simulink model "LAB3_CrazyFlie_2024_245678987654"  (R2023b)
settings: Solver=ode45  StartTime=0.0  StopTime=inf  MaxStep=0.1  RelTol=1e-3  EnableMultiTasking=on
PreLoadFcn:
  | % load parameters of the default quadrotor
  | disp('Quadrotor parameters loaded by PreLoadFcn')
  | mdl_quadrotor
values from neighbouring files (symbols this model uses):
  x = pos(:, 1)    [lab3_trajectory.m]    (also in plot.m = timeseries(x, time))
  y = pos(:, 2)    [lab3_trajectory.m]    (also in plot.m = timeseries(y, time))
  yaw = atan2(-y, -x)    [lab3_trajectory.m]    (also in plot.m = timeseries(yaw, time))
  z = pos(:, 3)    [lab3_trajectory.m]    (also in plot.m = timeseries(z, time))
undefined symbols (not defined in the file or in its folder): angdiff, Angular, Linear, rot2
libraries: robotlib x3, simulink x1
settings Model: Creator=corkep  LastModifiedBy=hampu
settings SolverCC: AlgebraicLoopSolver=TrustRegion
settings DataIOCC: LimitDataPoints=on  ReturnWorkspaceOutputs=off
settings OptimizationCC: ReuseModelBlockBuffer=off  ExpressionDepthLimit=2147483647  LifeSpan=inf
settings DebuggingCC: UnderspecifiedInitializationDetection=Classic  MergeDetectMultiDrivingBlocksExec=none  SolverPrmCheckMsg=warning  UnconnectedInputMsg=warning  UnconnectedOutputMsg=warning  UnconnectedLineMsg=warning  AllowSymbolicDim=off  StateNameClashWarn=warning  SFUnexpectedBacktrackingDiag=warning  SFNoUnconditionalDefaultTransitionDiag=warning  SFExecutionAtInitializationDiag=none  ArithmeticOperatorsInVariantConditions=warning
settings HardwareCC: ProdBitPerPointer=32  ProdBitPerSizeT=32  ProdBitPerPtrDiffT=32  ProdLargestAtomicFloat=None  ProdIntDivRoundTo=Undefined  ProdEndianess=Unspecified  ProdWordSize=32  ProdHWDeviceType=32-bit Generic
settings ModelReferenceCC: EnableRefExpFcnMdlSchedulingChecks=on  PropagateSignalLabelsOutOfModel=off
settings SFSimCC: SimUseLocalCustomCode=off  CustomCodeUndefinedFunction=UseInterfaceOnly
settings RTWCC: RTWUseLocalCustomCode=off  DLArmComputeVersion=19.05
settings CodeAppCC: StateflowObjectComments=on
settings GRTTargetCC: TargetLangStandard=C89/C90 (ANSI)  CombineOutputUpdateFcns=off  GRTInterface=on
settings ConfigComp: CovMetricSettings=dw  CovSaveCumulativeToWorkspaceVar=on  CovSaveSingleToWorkspaceVar=on  CovExternalEMLEnable=off  CovSFcnEnable=off

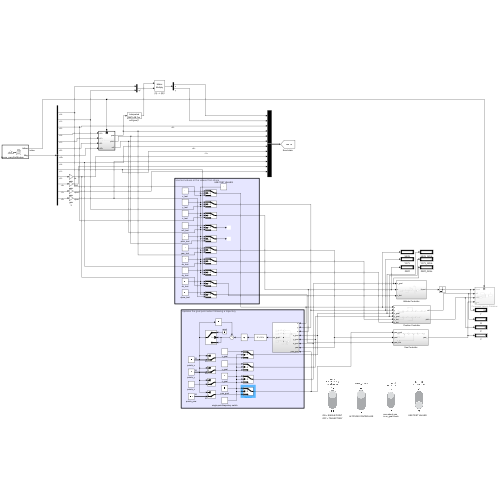
[thumbnail: Simulink's stored preview of the top-level diagram]
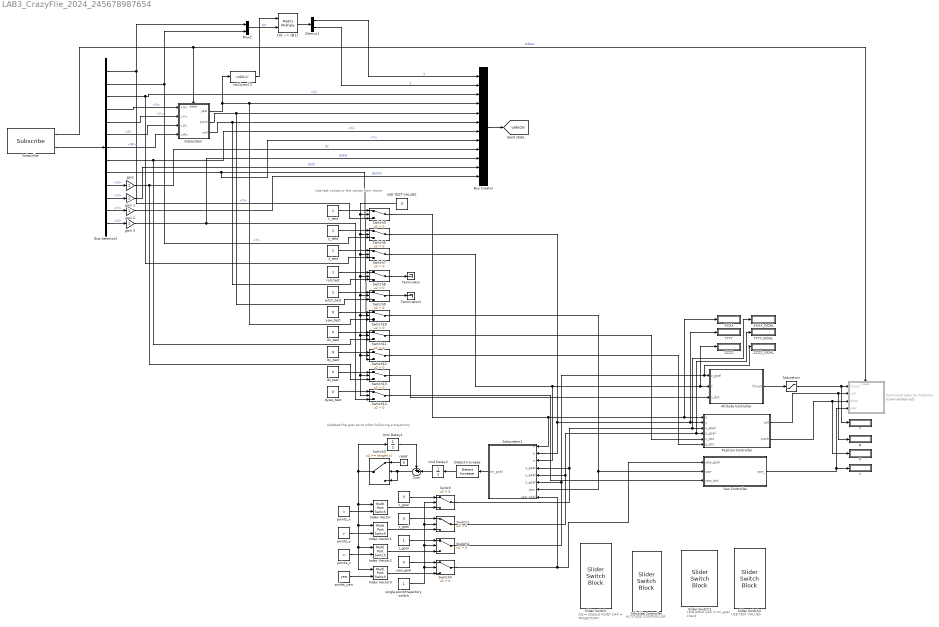
== system LAB3_CrazyFlie_2024_245678987654 ==
  note: Use test values or the values from drone
  note: USE TEST VALUES
  note: care about yaw
      | in on_goal check
  note: ON = SINGLE POINT
      | OFF = TRAJECTORY
  note: Updates the goal point when following a trajectory
  note: ALTITUDE CONTROLLER
  Altitude Controller : Subsystem
  Altiutide Controller : SliderSwitchBlock
      settings: Values={{'Off', 'On'}, [0 1]}
  Bus Creator : BusCreator  Inputs=12
  Bus Selector3 : BusSelector  OutputSignals=Pose.Pose.Position.X,Pose.Pose.Position.Y,Pose.Pose.Position.Z,Pose.Pose.Orientation.X,Pose.Pose.Orientation.Y,Pose.Pose.Orientation.Z,Pose.Pose.Orientation.W,Twist.Twist.Linear.X,Twist.Twist.Linear.Y,Twist.Twist.Linear.Z,Twist.Twist.Angular.X,Twist.Twist.Angular.Y,Twist.Twist.Angular.Z
  Command Velocity Publisher : Subsystem  Commented=on
  Demux1 : Demux  Outputs=2
  Detect Increase : simulink/Logic and Bit Operations/Detect Increase  vinit=0.0  OutDataTypeStr=boolean
  Index Vector{,1..3} (4 alike) : MultiPortSwitch  DataPortOrder=Zero-based contiguous  Inputs=1  zeroidx=on  SaturateOnIntegerOverflow=off  InputSameDT=off
  Mux2 : Mux  Inputs=2
  P : Display
  Position Controller : Subsystem
  R : Display
  Saturation : Saturate  UpperLimit=1  LowerLimit=0
  Slider Switch : SliderSwitchBlock
      settings: Values={{'Off', 'On'}, [0 1]}
  Slider Switch1 : SliderSwitchBlock
      settings: Values={{'Off', 'On'}, [0 1]}
  Slider Switch2 : SliderSwitchBlock
      settings: Values={{'Off', 'On'}, [0 1]}
  Subscribe : robotlib/Subscribe  topicSource=Select from ROS network  topic=/pixy/vicon/demo_crazyflie28/demo_crazyflie28/odom  messageType=nav_msgs/Odometry  SampleTime=-1  legacyBusStruct=off  messageQueueLength=51
  Subsystem : Subsystem
  Subsystem1 : Subsystem
  Sum : Sum  Inputs=++|
  Switch{,1..2,4..14} (14 alike) : Switch  Criteria=u2 > Threshold  SaturateOnIntegerOverflow=off  InputSameDT=off
  Switch3 : Switch  Threshold=length(x)  SaturateOnIntegerOverflow=off  InputSameDT=off
  T : Display
  Terminator : Terminator
  Terminator1 : Terminator
  USE TEST VALUES : Constant  Value=0
  Unit Delay2 : UnitDelay  SampleTime=-1  HasFrameUpgradeWarning=on
  Unit Delay4 : UnitDelay  SampleTime=-1  HasFrameUpgradeWarning=on
  XXXX : Display
  XXXX_GOAL : Display
  Y : Display
  YYYY : Display
  YYYY_GOAL : Display
  Yaw Controller : Subsystem
  ZZZZ : Display
  ZZZZ_GOAL : Display
  dx_test : Constant  Value=0
  dy_test : Constant  Value=0
  dyaw_test : Constant  Value=0
  dz_test : Constant  Value=0
  gain {,1..3} (4 alike) : Gain
  pitch_test : Constant
  points_x : Constant  Value=x
  points_y : Constant  Value=y
  points_yaw : Constant  Value=yaw
  points_z : Constant  Value=z
  reset : Constant  Value=0  VectorParams1D=off
  roll_test : Constant
  rot2(yaw)'1 : MATLABFcn  MATLABFcn=rot2(u)'  OutputDimensions=[2 2]  Output1D=off
  single point/trajectory switch : Constant
  x_goal : Constant  Value=3
  x_test : Constant
  y_goal : Constant  Value=3
  y_test : Constant
  yaw_goal : Constant  Value=0
  yaw_test : Constant  Value=0
  z_goal : Constant
  z_test : Constant
  "{0} --> {B}1" : Product  Multiplication=Matrix(*)  RndMeth=Zero
  tag scope: vehicle=global
  wires:
  Bus Selector3/11 -> gain 1/1  "<X>"
  Bus Selector3/13 -> gain 3/1  "<Z>"
  Bus Selector3/10 -> "gain "/1  "<Z>"
  Bus Selector3/9 -> Switch12/3, Bus Creator/8  "<Y>"
  Bus Selector3/8 -> Switch11/3, Bus Creator/7  "<X>"
  Bus Selector3/3 -> Switch7/3, Bus Creator/3  "<Z>"
  Bus Creator/1 -> [vehicle]
  Bus Selector3/12 -> gain 2/1  "<Y>"
  Subscribe/2 -> Bus Selector3/1
  Subscribe/1 -> Subsystem/Enable, Command Velocity Publisher/Enable  "IsNew"
  Mux2/1 -> "{0} --> {B}1"/2  "xy*"
  "{0} --> {B}1"/1 -> Demux1/1
  Demux1/1 -> Bus Creator/1  "x"
  Demux1/2 -> Bus Creator/2  "y"
  Bus Selector3/1 -> Mux2/1, Switch5/3  "<X>"
  Bus Selector3/2 -> Switch6/3, Mux2/2  "<Y>"
  rot2(yaw)'1/1 -> "{0} --> {B}1"/1
  "gain "/1 -> Switch13/3, Bus Creator/9  "dz"
  gain 1/1 -> Bus Creator/11  "droll"
  gain 2/1 -> Bus Creator/12  "dpitch"
  gain 3/1 -> Switch14/3, Bus Creator/10  "dyaw"
  Subsystem/1(yaw) -> rot2(yaw)'1/1, Switch10/3, Bus Creator/4
  Bus Selector3/4 -> Subsystem/1(<X>)  "<X>"
  Bus Selector3/5 -> Subsystem/2(<Y>)  "<Y>"
  Bus Selector3/6 -> Subsystem/3(<Z>)  "<Z>"
  Bus Selector3/7 -> Subsystem/4(<W>)  "<W>"
  Subsystem/2(pitch) -> Switch9/3, Bus Creator/5
  Subsystem/3(roll) -> Switch8/3, Bus Creator/6
  Altitude Controller/1(thrust) -> Saturation/1
  Saturation/1 -> T/1, Command Velocity Publisher/1(thrust)
  x_goal/1 -> Switch/1
  Position Controller/2(pitch) -> P/1, Command Velocity Publisher/3(pitch)
  Position Controller/1(roll) -> R/1, Command Velocity Publisher/2(roll)
  Yaw Controller/1(yaw_) -> Command Velocity Publisher/4(yaw), Y/1
  Unit Delay4/1 -> Sum/1
  Sum/1 -> Switch3/3, Switch3/2
  Unit Delay2/1 -> Sum/2
  Switch3/1 -> Index Vector3/1, Index Vector2/1, Index Vector1/1, Index Vector/1, Unit Delay4/1
  reset/1 -> Switch3/1
  Detect Increase/1 -> Unit Delay2/1
  Subsystem1/1(on_goal) -> Detect Increase/1
  points_x/1 -> Index Vector/2
  points_y/1 -> Index Vector1/2
  points_z/1 -> Index Vector2/2
  points_yaw/1 -> Index Vector3/2
  Switch/1 -> XXXX_GOAL/1, Position Controller/3(x_goal), Subsystem1/4(x_goal)
  Index Vector/1 -> Switch/3
  Index Vector1/1 -> Switch1/3
  Index Vector2/1 -> Switch2/3
  Index Vector3/1 -> Switch4/3
  y_goal/1 -> Switch1/1
  z_goal/1 -> Switch2/1
  yaw_goal/1 -> Switch4/1
  single point/trajectory switch/1 -> Switch/2, Switch1/2, Switch2/2, Switch4/2
  Switch4/1 -> Subsystem1/8(yaw_goal), Yaw Controller/1(yaw_goal)
  Switch2/1 -> ZZZZ_GOAL/1, Altitude Controller/1(z_goal), Subsystem1/6(z_goal)
  Switch1/1 -> YYYY_GOAL/1, Position Controller/4(y_goal), Subsystem1/5(y_goal)
  x_test/1 -> Switch5/1
  y_test/1 -> Switch6/1
  z_test/1 -> Switch7/1
  USE TEST VALUES/1 -> Switch14/2, Switch13/2, Switch12/2, Switch11/2, Switch10/2, Switch9/2, Switch8/2, Switch7/2, Switch6/2, Switch5/2
  roll_test/1 -> Switch8/1
  pitch_test/1 -> Switch9/1
  yaw_test/1 -> Switch10/1
  dx_test/1 -> Switch11/1
  dy_test/1 -> Switch12/1
  dz_test/1 -> Switch13/1
  dyaw_test/1 -> Switch14/1
  Switch7/1 -> Subsystem1/3(z), ZZZZ/1, Altitude Controller/2(z)
  Switch5/1 -> XXXX/1, Position Controller/1(x), Subsystem1/1(x)
  Switch6/1 -> YYYY/1, Position Controller/2(y), Subsystem1/2(y)
  Switch8/1 -> Terminator/1
  Switch10/1 -> Subsystem1/7(yaw), Yaw Controller/2(yaw)
  Switch11/1 -> Position Controller/5(x_dot)
  Switch12/1 -> Position Controller/6(y_dot)
  Switch13/1 -> Altitude Controller/3(z_dot)
  Switch14/1 -> Yaw Controller/3(yaw_dot)
  Switch9/1 -> Terminator1/1

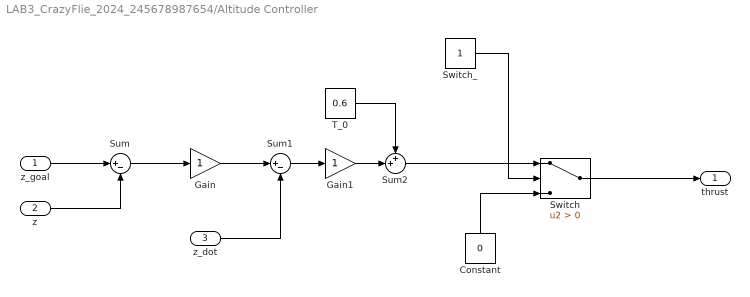
== system LAB3_CrazyFlie_2024_245678987654/Altitude Controller ==
  z_goal : Inport
  z : Inport  Port=2
  z_dot : Inport  Port=3
  Constant : Constant  Value=0
  Gain : Gain
  Gain1 : Gain
  Sum : Sum  Inputs=|+-
  Sum1 : Sum  Inputs=|+-
  Sum2 : Sum  Inputs=++|
  Switch : Switch  Criteria=u2 > Threshold  SaturateOnIntegerOverflow=off  InputSameDT=off
  Switch_ : Constant
  T_0 : Constant  Value=0.6
  thrust : Outport
  wires:
  z_goal/1 -> Sum/1
  z/1 -> Sum/2
  Sum2/1 -> Switch/1
  Switch/1 -> thrust/1
  Constant/1 -> Switch/3
  Switch_/1 -> Switch/2
  Sum/1 -> Gain/1
  Gain1/1 -> Sum2/2
  Sum1/1 -> Gain1/1
  T_0/1 -> Sum2/1
  Gain/1 -> Sum1/1
  z_dot/1 -> Sum1/2

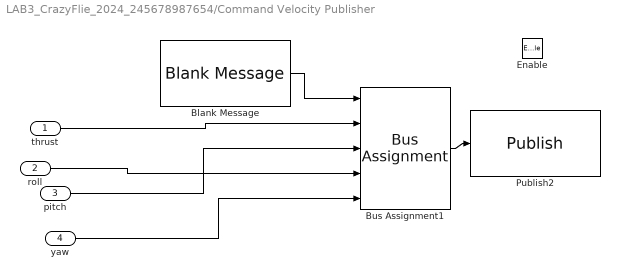
== system LAB3_CrazyFlie_2024_245678987654/Command Velocity Publisher ==
  thrust : Inport
  roll : Inport  Port=2
  pitch : Inport  Port=3
  yaw : Inport  Port=4
  Enable : EnablePort
  Blank Message : robotlib/Blank Message  messageClass=Message  entityType=geometry_msgs/Twist  messageType=geometry_msgs/Twist  SampleTime=inf  legacyBusStruct=off
  Bus Assignment1 : BusAssignment  DialogController=Simulink.DDGSource_BusAssignment  AssignedSignals=Linear.Z,Linear.X,Linear.Y,Angular.Z
  Publish2 : robotlib/Publish  topicSource=Select from ROS network  topic=/demo_crazyflie3/cmd_vel  messageType=geometry_msgs/Twist  legacyBusStruct=off  messageQueueLength=105
  wires:
  Bus Assignment1/1 -> Publish2/1
  Blank Message/1 -> Bus Assignment1/1
  yaw/1 -> Bus Assignment1/5
  roll/1 -> Bus Assignment1/4
  pitch/1 -> Bus Assignment1/3
  thrust/1 -> Bus Assignment1/2

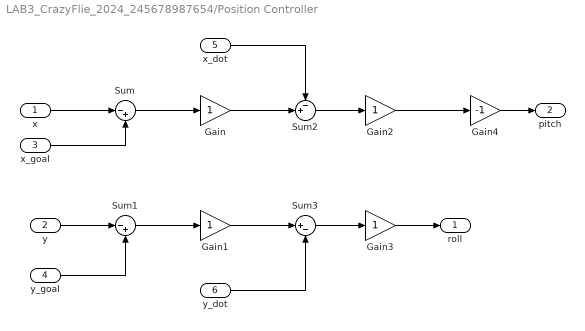
== system LAB3_CrazyFlie_2024_245678987654/Position Controller ==
  x : Inport
  y : Inport  Port=2
  x_goal : Inport  Port=3
  y_goal : Inport  Port=4
  x_dot : Inport  Port=5
  y_dot : Inport  Port=6
  Gain{,1..3} (4 alike) : Gain
  Gain4 : Gain  Gain=-1
  Sum : Sum  Inputs=|-+
  Sum1 : Sum  Inputs=|-+
  Sum2 : Sum  Inputs=-+|
  Sum3 : Sum  Inputs=|+-
  roll : Outport
  pitch : Outport  Port=2
  wires:
  y/1 -> Sum1/1
  y_goal/1 -> Sum1/2
  x/1 -> Sum/1
  x_goal/1 -> Sum/2
  Sum/1 -> Gain/1
  Sum1/1 -> Gain1/1
  Gain1/1 -> Sum3/1
  Gain/1 -> Sum2/2
  x_dot/1 -> Sum2/1
  y_dot/1 -> Sum3/2
  Sum3/1 -> Gain3/1
  Sum2/1 -> Gain2/1
  Gain2/1 -> Gain4/1
  Gain3/1 -> roll/1
  Gain4/1 -> pitch/1

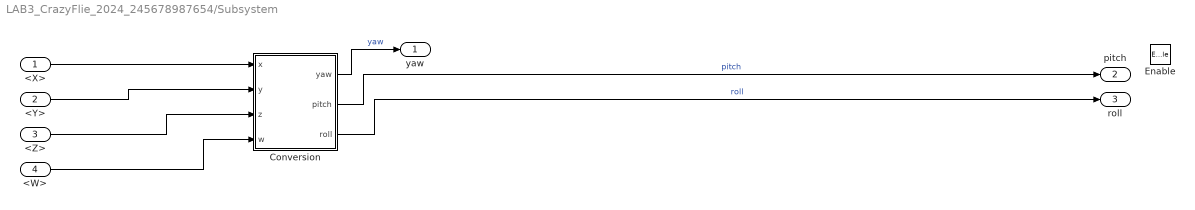
== system LAB3_CrazyFlie_2024_245678987654/Subsystem ==
  <X> : Inport
  <Y> : Inport  Port=2
  <Z> : Inport  Port=3
  <W> : Inport  Port=4
  Enable : EnablePort
  Conversion : MATLAB Function  TreatAsAtomicUnit=on
  yaw : Outport
  pitch : Outport  Port=2
  roll : Outport  Port=3
  wires:
  Conversion/1(yaw) -> yaw/1  "yaw"
  <X>/1 -> Conversion/1(x)
  Conversion/2(pitch) -> pitch/1  "pitch"
  <W>/1 -> Conversion/4(w)
  <Y>/1 -> Conversion/2(y)
  Conversion/3(roll) -> roll/1  "roll"
  <Z>/1 -> Conversion/3(z)

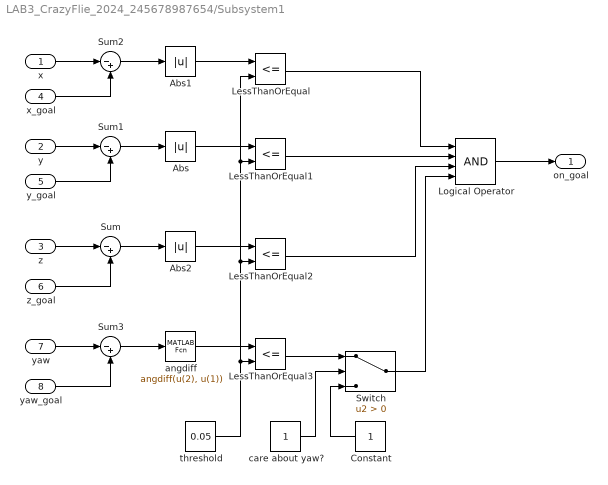
== system LAB3_CrazyFlie_2024_245678987654/Subsystem1 ==
  x : Inport
  y : Inport  Port=2
  z : Inport  Port=3
  x_goal : Inport  Port=4
  y_goal : Inport  Port=5
  z_goal : Inport  Port=6
  yaw : Inport  Port=7
  yaw_goal : Inport  Port=8
  Abs : Abs  SaturateOnIntegerOverflow=off
  Abs1 : Abs  SaturateOnIntegerOverflow=off
  Abs2 : Abs  SaturateOnIntegerOverflow=off
  Constant : Constant
  LessThanOrEqual{,1..3} (4 alike) : RelationalOperator  Operator=<=  OutDataTypeStr=boolean  RndMeth=Simplest  InputSameDT=off
  Logical Operator : Logic  Inputs=4  AllPortsSameDT=off  OutDataTypeStr=boolean
  Sum{,1..3} (4 alike) : Sum  Inputs=|-+
  Switch : Switch  Criteria=u2 > Threshold  SaturateOnIntegerOverflow=off  InputSameDT=off
  angdiff : MATLABFcn  MATLABFcn=angdiff(u(2), u(1))
  care about yaw? : Constant
  threshold : Constant  Value=0.05
  on_goal : Outport
  wires:
  z/1 -> Sum/1
  y/1 -> Sum1/1
  x/1 -> Sum2/1
  x_goal/1 -> Sum2/2
  y_goal/1 -> Sum1/2
  z_goal/1 -> Sum/2
  Sum2/1 -> Abs1/1
  Sum1/1 -> Abs/1
  Sum/1 -> Abs2/1
  Logical Operator/1 -> on_goal/1
  Abs1/1 -> LessThanOrEqual/1
  Abs/1 -> LessThanOrEqual1/1
  Abs2/1 -> LessThanOrEqual2/1
  threshold/1 -> LessThanOrEqual3/2, LessThanOrEqual/2, LessThanOrEqual1/2, LessThanOrEqual2/2
  LessThanOrEqual/1 -> Logical Operator/1
  LessThanOrEqual1/1 -> Logical Operator/2
  LessThanOrEqual2/1 -> Logical Operator/3
  yaw_goal/1 -> Sum3/2
  yaw/1 -> Sum3/1
  Sum3/1 -> angdiff/1
  angdiff/1 -> LessThanOrEqual3/1
  Constant/1 -> Switch/3
  LessThanOrEqual3/1 -> Switch/1
  Switch/1 -> Logical Operator/4
  care about yaw?/1 -> Switch/2

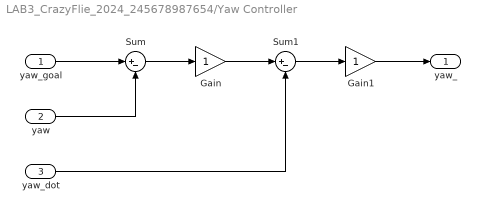
== system LAB3_CrazyFlie_2024_245678987654/Yaw Controller ==
  yaw_goal : Inport
  yaw : Inport  Port=2
  yaw_dot : Inport  Port=3
  Gain : Gain
  Gain1 : Gain
  Sum : Sum  Inputs=|+-
  Sum1 : Sum  Inputs=|+-
  yaw_ : Outport
  wires:
  yaw_goal/1 -> Sum/1
  yaw/1 -> Sum/2
  Sum/1 -> Gain/1
  Gain/1 -> Sum1/1
  Sum1/1 -> Gain1/1
  Gain1/1 -> yaw_/1
  yaw_dot/1 -> Sum1/2

== matlab function LAB3_CrazyFlie_2024_245678987654/Subsystem/Conversion ==
  data: yaw output; x input; y input; z input; w input; pitch output; roll output
function [yaw,pitch,roll]  = quat2eul(x,y,z,w)
%#codegen

% Convert the quaternion to a yaw angle (zyx euler angle)
eul = quat2eul([w,x,y,z]);
yaw = eul(1);
roll = eul(3);
pitch = eul(2);

end
